simulink model "lookupTableDynamic_TestGen32"  (R2017b)
settings: Solver=FixedStepDiscrete  StartTime=0.0  StopTime=10.0  RelTol=1e-3
undefined symbols (not defined in the file): Block_TestLib, enable_trigger
libraries: simulink x1
settings Model: Creator=ktrinh  LastModifiedBy=ktrinh
settings DebuggingCC: ParameterOverflowMsg=none

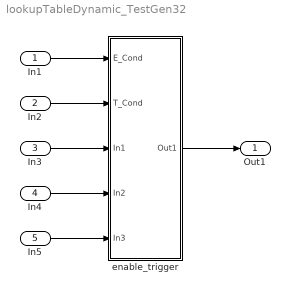
== system lookupTableDynamic_TestGen32 ==
  In1 : Inport
  In2 : Inport  Port=2
  In3 : Inport  Port=3
  In4 : Inport  Port=4
  In5 : Inport  Port=5
  enable_trigger : Subsystem  AncestorBlock=Block_TestLib/enable_trigger
  Out1 : Outport
  wires:
  In1/1 -> enable_trigger/1(E_Cond)
  In2/1 -> enable_trigger/2(T_Cond)
  In3/1 -> enable_trigger/3(In1)
  In4/1 -> enable_trigger/4(In2)
  In5/1 -> enable_trigger/5(In3)
  enable_trigger/1(Out1) -> Out1/1

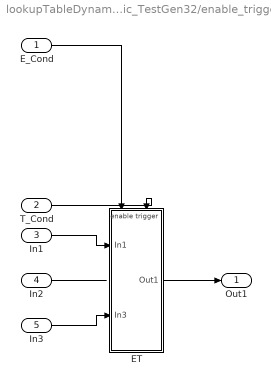
== system lookupTableDynamic_TestGen32/enable_trigger ==
  E_Cond : Inport  OutDataTypeStr=boolean
  T_Cond : Inport  Port=2  OutDataTypeStr=boolean
  In1 : Inport  Port=3
  In2 : Inport  Port=4
  In3 : Inport  Port=5
  ET : Subsystem  TreatAsAtomicUnit=on
  Out1 : Outport
  wires:
  T_Cond/1 -> ET/Trigger
  E_Cond/1 -> ET/Enable
  In1/1 -> ET/1(In1)
  In2/1 -> ?
  In3/1 -> ET/2(In3)
  ET/1(Out1) -> Out1/1

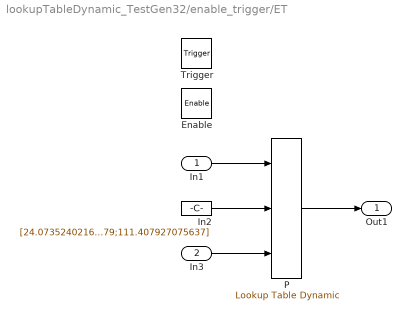
== system lookupTableDynamic_TestGen32/enable_trigger/ET ==
  In1 : Inport  OutMin=22.0735  OutMax=113  OutDataTypeStr=uint32  PortDimensions=1
  In3 : Inport  Port=2  PortDimensions=5
  Enable : EnablePort
  Trigger : TriggerPort  VariantControl=Variant
  In2 : Constant  Value=[24.073524021666;55.8575959338135;60.8681056881964;63.1673304299079;111.407927075637]  OutDataTypeStr=uint32
  P : simulink/Lookup Tables/Lookup Table Dynamic  LookUpMeth=Use Input Below  OutDataType=fixdt('int16')  OutScaling=[]  OutputDataTypeScalingMode=Specify via dialog  OutDataTypeStr=int16  RndMeth=Round  DoSatur=off
      settings: SourceProductName=Simulink
  Out1 : Outport
  wires:
  In1/1 -> P/1
  In2/1 -> P/2
  In3/1 -> P/3
  P/1 -> Out1/1
